simulink model "scenario"  (R2022a)
settings: Solver=FixedStepDiscrete  StartTime=0.0  StopTime=200  RelTol=1e-3
model workspace (MAT data in the model file):
  firstWarning = 1
  originalScenarioChecksum = '4DD51816F7E71EE9C2F131BDCC6CE010'
undefined symbols (not defined in the file or in its folder): driving
libraries: drivingscenarioandsensors x4
settings Model: Creator=giovanni02  LastModifiedBy=giovanni02

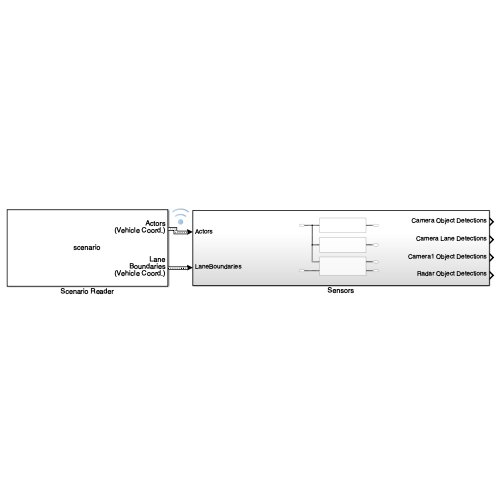
[thumbnail: Simulink's stored preview of the top-level diagram]
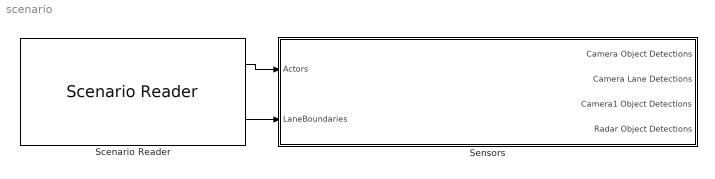
== system scenario ==
  Scenario Reader : drivingscenarioandsensors/Scenario Reader  ScenarioSource=From file  ScenarioFileName=/Users/giovanni02/Desktop/Progetti/HybridRL/scenario.mat  ScenarioVariableName=scenario  OutputCoordinateSystem=Vehicle coordinates  EgoVehicleSource=Scenario  EgoVehicleActorID=1  OrientVehiclesOnRoad=off  OutputEgoVehiclePose=off  OutputEgoVehicleState=off  SampleTime=0.1  LaneBoundaryOutput=Ego vehicle lane boundaries  LaneBoundaryDistance=linspace(-150, 150, 101)  LaneBoundaryLocation=Center of lane markings  BusNameSource=Auto  BusName=BusActors  BusNumActorsSource=Scenario  BusNumActors=100  BusName2Source=Auto  BusName2=BusLaneBoundaries  BusNumLaneBoundariesSource=Scenario  BusNumLaneBoundaries=10  BusName3Source=Auto  BusName3=BusEgoActor  BusName4Source=Auto  BusName4=BusEgoState  ShowCoordinateLabels=on  SimulateUsing=Interpreted execution
  Sensors : Subsystem
  wires:
  Scenario Reader/1 -> Sensors/1(Actors)
  Scenario Reader/2 -> Sensors/2(LaneBoundaries)

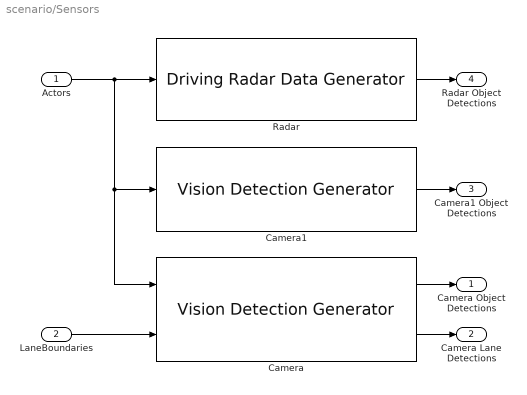
== system scenario/Sensors ==
  Actors : Inport
  LaneBoundaries : Inport  Port=2
  Camera : drivingscenarioandsensors/Vision Detection Generator  SensorIndex=1  DetectorOutput=Lanes and objects  UpdateInterval=0.1  LaneUpdateInterval=0.1  SensorLocation=[1.9 0]  Height=1.1  Yaw=0  Pitch=1  Roll=0  BusNameSource=Auto  BusName=BusObjectDetections  BusName2Source=Auto  BusName2=BusLaneDetections  MaxNumDetectionsSource=Property  MaxNumDetections=50  MaxNumLanesSource=Property  MaxNumLanes=30  DetectionCoordinates=Ego Cartesian  SimulateUsing=Interpreted execution  MaxRange=150  BoundingBoxAccuracy=5  ProcessNoiseIntensity=5  MaxSpeed=100  MaxAllowedOcclusion=0.5  MinObjectImageSize=[15 15]  DetectionProbability=0.9  FalsePositivesPerImage=0.1  MinLaneImageSize=[20 3]  LaneBoundaryAccuracy=3  HasNoise=on  InitialSeedSource=Repeatable  InitialSeed=0  UsedSeed=0  ActorProfilesSource=From Scenario Reader block  ActorProfilesParameters=driving.internal.ActorProfilesParameters  ActorProfilesExpression=[struct('ActorID',1,'ClassID',1,'Length',4.848,'Width',1.842,'Height',1.517,'OriginOffset',[-1.305 0 0],'MeshVertices',[3.729 0.921 0.929096885813149;3.729 -0.921 0.929096885813149;3.729 -0.921 0.341193771626297;3.729 0.921 0.341193771626297;3.729 0.921 0.929096885813149;2.517 0.921 1.07607266435986;2.517 -0.921 1.07607266435986;3.729 -0.921 0.929096885813149;1.7898 0.7368 1.517;0.3354 0.7368 1.517;0.3354 -0.7368 1.517;1.7898 -0.7368 1.517;-0.3918 0.921 1.07607266435986;-1.119 0.921 0.929096885813149;-1.119 -0.921 0.929096885813149;-0.3918 -0.921 1.07607266435986;3.729 0.921 0.929096885813149;3.729 0.921 0.341193771626297;2.517 0.921 0.341193771626297;2.517 0.921 1.07607266435986;2.517 0.921 1.07607266435986;2.517 0.921 0.341193771626297;-0.3918 0.921 0.341193771626297;-0.3918 0.921 1.07607266435986;-0.3918 0.921 1.07607266435986;-0.3918 0.921 0.341193771626297;-1.119 0.921 0.385286505190311;-1.119 0.921 0.929096885813149;2.517 0.921 1.07607266435986;-0.3918 0.921 1.07607266435986;0.3354 0.7368 1.517;1.7898 0.7368 1.517;3.729 -0.921 0.929096885813149;3.729 -0.921 0.341193771626297;2.517 -0.921 0.341193771626297;2.517 -0.921 1.07607266435986;2.517 -0.921 1.07607266435986;2.517 -0.921 0.341193771626297;-0.3918 -0.921 0.341193771626297;-0.3918 -0.921 1.07607266435986;-0.3918 -0.921 1.07607266435986;-0.3918 -0.921 0.341193771626297;-1.119 -0.921 0.385286505190311;-1.119 -0.921 0.929096885813149;2.517 -0.921 1.07607266435986;-0.3918 -0.921 1.07607266435986;0.3354 -0.7368 1.517;1.7898 -0.7368 1.517;-0.3918 0.921 1.07607266435986;-0.3918 -0.921 1.07607266435986;0.3354 -0.7368 1.517;0.3354 0.7368 1.517;2.517 -0.921 1.07607266435986;1.7898 -0.7368 1.517;1.7898 0.7368 1.517;2.517 0.921 1.07607266435986;-1.119 0.921 0.929096885813149;-1.119 0.921 0.385286505190311;-1.119 -0.921 0.385286505190311;-1.119 -0.921 0.929096885813149;3.729 0.921 0.341193771626297;3.729 -0.921 0.341193771626297;-0.3918 -0.921 0.341193771626297;-0.3918 0.921 0.341193771626297;-0.3918 0.921 0.341193771626297;-1.119 0.921 0.385286505190311;-1.119 -0.921 0.385286505190311;-0.3918 -0.921 0.341193771626297;-0.0875106382978725 -0.6447 0;-0.0875106382978725 -0.8903 0;0.109534987981281 -0.6447 0.065162212005738;0.109534987981281 -0.8903 0.065162212005738;0.231315882356307 -0.6447 0.235759097818887;0.231315882356307 -0.8903 0.235759097818887;0.231315882356307 -0.6447 0.446628445433708;0.231315882356307 -0.8903 0.446628445433708;0.109534987981281 -0.6447 0.617225331246857;0.109534987981281 -0.8903 0.617225331246857;-0.0875106382978725 -0.6447 0.682387543252595;-0.0875106382978725 -0.8903 0.682387543252595;-0.284556264577026 -0.6447 0.617225331246857;-0.284556264577026 -0.8903 0.617225331246857;-0.406337158952052 -0.6447 0.446628445433708;-0.406337158952052 -0.8903 0.446628445433708;-0.406337158952052 -0.6447 0.235759097818887;-0.406337158952052 -0.8903 0.235759097818887;-0.284556264577026 -0.6447 0.065162212005738;-0.284556264577026 -0.8903 0.065162212005738;-0.0875106382978725 -0.6447 0;-0.0875106382978725 -0.8903 0;-0.0875106382978725 -0.6447 0;0.109534987981281 -0.6447 0.065162212005738;0.231315882356307 -0.6447 0.235759097818887;0.231315882356307 -0.6447 0.446628445433708;0.109534987981281 -0.6447 0.617225331246857;-0.0875106382978725 -0.6447 0.682387543252595;-0.284556264577026 -0.6447 0.617225331246857;-0.406337158952052 -0.6447 0.446628445433708;-0.406337158952052 -0.6447 0.235759097818887;-0.284556264577026 -0.6447 0.065162212005738;-0.0875106382978725 -0.8903 0;0.109534987981281 -0.8903 0.065162212005738;0.231315882356307 -0.8903 0.235759097818887;0.231315882356307 -0.8903 0.446628445433708;0.109534987981281 -0.8903 0.617225331246857;-0.0875106382978725 -0.8903 0.682387543252595;-0.284556264577026 -0.8903 0.617225331246857;-0.406337158952052 -0.8903 0.446628445433708;-0.406337158952052 -0.8903 0.235759097818887;-0.284556264577026 -0.8903 0.065162212005738;-0.0875106382978725 0.8903 0;-0.0875106382978725 0.6447 0;0.109534987981281 0.8903 0.065162212005738;0.109534987981281 0.6447 0.065162212005738;0.231315882356307 0.8903 0.235759097818887;0.231315882356307 0.6447 ...(+4912 chars)],'MeshFaces',[1 2 3;3 4 1;5 6 7;7 8 5;9 10 11;11 12 9;13 14 15;15 16 13;17 18 19;19 20 17;21 22 23;23 24 21;25 26 27;27 28 25;29 30 31;31 32 29;33 34 35;35 36 33;37 38 39;39 40 37;41 42 43;43 44 41;45 46 47;47 48 45;49 50 51;51 52 49;53 54 55;55 56 53;57 58 59;59 60 57;61 62 63;63 64 61;65 66 67;67 68 65;69 71 72;72 70 69;71 73 74;74 72 71;73 75 76;76 74 73;75 77 78;78 76 75;77 79 80;80 78 77;79 81 82;82 80 79;81 83 84;84 82 81;83 85 86;86 84 83;85 87 88;88 86 85;87 89 90;90 88 87;91 92 93;91 93 94;91 94 95;91 95 96;91 96 97;91 97 98;91 98 99;91 99 100;101 102 103;101 103 104;101 104 105;101 105 106;101 106 107;101 107 108;101 108 109;101 109 110;111 113 114;114 112 111;113 115 116;116 114 113;115 117 118;118 116 115;117 119 120;120 118 117;119 121 122;122 120 119;121 123 124;124 122 121;123 125 126;126 124 123;125 127 128;128 126 125;127 129 130;130 128 127;129 131 132;132 130 129;133 134 135;133 135 136;133 136 137;133 137 138;133 138 139;133 139 140;133 140 141;133 141 142;143 144 145;143 145 146;143 146 147;143 147 148;143 148 149;143 149 150;143 150 151;143 151 152;153 155 156;156 154 153;155 157 158;158 156 155;157 159 160;160 158 157;159 161 162;162 160 159;161 163 164;164 162 161;163 165 166;166 164 163;165 167 168;168 166 165;167 169 170;170 168 167;169 171 172;172 170 169;171 173 174;174 172 171;175 176 177;175 177 178;175 178 179;175 179 180;175 180 181;175 181 182;175 182 183;175 183 184;185 186 187;185 187 188;185 188 189;185 189 190;185 190 191;185 191 192;185 192 193;185 193 194;195 197 198;198 196 195;197 199 200;200 198 197;199 201 202;202 200 199;201 203 204;204 202 201;203 205 206;206 204 203;205 207 208;208 206 205;207 209 210;210 208 207;209 211 212;212 210 209;211 213 214;214 212 211;213 215 216;216 214 213;217 218 219;217 219 220;217 220 221;217 221 222;217 222 223;217 223 224;217 224 225;217 225 226;227 228 229;227 229 230;227 230 231;227 231 232;227 232 233;227 233 234;227 234 235;227 235 236],'RCSPattern',[10 10;10 10],'RCSAzimuthAngles',[-180 180],'RCSElevationAngles',[-90 90])]  Intrinsics=driving.internal.cameraIntrinsics('FocalLength',[800 800],'PrincipalPoint',[400 240],'ImageSize',[500 700],'RadialDistortion',[0 0],'TangentialDistortion',[0 0],'Skew',0)
  Camera1 : drivingscenarioandsensors/Vision Detection Generator  SensorIndex=2  DetectorOutput=Objects only  UpdateInterval=0.1  LaneUpdateInterval=0.1  SensorLocation=[-1 0]  Height=1.1  Yaw=-180  Pitch=1  Roll=0  BusNameSource=Auto  BusName=BusObjectDetections  BusName2Source=Auto  BusName2=BusLaneDetections  MaxNumDetectionsSource=Property  MaxNumDetections=50  MaxNumLanesSource=Property  MaxNumLanes=30  DetectionCoordinates=Ego Cartesian  SimulateUsing=Interpreted execution  MaxRange=100  BoundingBoxAccuracy=5  ProcessNoiseIntensity=5  MaxSpeed=100  MaxAllowedOcclusion=0.5  MinObjectImageSize=[15 15]  DetectionProbability=0.9  FalsePositivesPerImage=0.1  MinLaneImageSize=[20 3]  LaneBoundaryAccuracy=3  HasNoise=on  InitialSeedSource=Repeatable  InitialSeed=0  UsedSeed=0  ActorProfilesSource=From Scenario Reader block  ActorProfilesParameters=driving.internal.ActorProfilesParameters  ActorProfilesExpression=[struct('ActorID',1,'ClassID',1,'Length',4.848,'Width',1.842,'Height',1.517,'OriginOffset',[-1.305 0 0],'MeshVertices',[3.729 0.921 0.929096885813149;3.729 -0.921 0.929096885813149;3.729 -0.921 0.341193771626297;3.729 0.921 0.341193771626297;3.729 0.921 0.929096885813149;2.517 0.921 1.07607266435986;2.517 -0.921 1.07607266435986;3.729 -0.921 0.929096885813149;1.7898 0.7368 1.517;0.3354 0.7368 1.517;0.3354 -0.7368 1.517;1.7898 -0.7368 1.517;-0.3918 0.921 1.07607266435986;-1.119 0.921 0.929096885813149;-1.119 -0.921 0.929096885813149;-0.3918 -0.921 1.07607266435986;3.729 0.921 0.929096885813149;3.729 0.921 0.341193771626297;2.517 0.921 0.341193771626297;2.517 0.921 1.07607266435986;2.517 0.921 1.07607266435986;2.517 0.921 0.341193771626297;-0.3918 0.921 0.341193771626297;-0.3918 0.921 1.07607266435986;-0.3918 0.921 1.07607266435986;-0.3918 0.921 0.341193771626297;-1.119 0.921 0.385286505190311;-1.119 0.921 0.929096885813149;2.517 0.921 1.07607266435986;-0.3918 0.921 1.07607266435986;0.3354 0.7368 1.517;1.7898 0.7368 1.517;3.729 -0.921 0.929096885813149;3.729 -0.921 0.341193771626297;2.517 -0.921 0.341193771626297;2.517 -0.921 1.07607266435986;2.517 -0.921 1.07607266435986;2.517 -0.921 0.341193771626297;-0.3918 -0.921 0.341193771626297;-0.3918 -0.921 1.07607266435986;-0.3918 -0.921 1.07607266435986;-0.3918 -0.921 0.341193771626297;-1.119 -0.921 0.385286505190311;-1.119 -0.921 0.929096885813149;2.517 -0.921 1.07607266435986;-0.3918 -0.921 1.07607266435986;0.3354 -0.7368 1.517;1.7898 -0.7368 1.517;-0.3918 0.921 1.07607266435986;-0.3918 -0.921 1.07607266435986;0.3354 -0.7368 1.517;0.3354 0.7368 1.517;2.517 -0.921 1.07607266435986;1.7898 -0.7368 1.517;1.7898 0.7368 1.517;2.517 0.921 1.07607266435986;-1.119 0.921 0.929096885813149;-1.119 0.921 0.385286505190311;-1.119 -0.921 0.385286505190311;-1.119 -0.921 0.929096885813149;3.729 0.921 0.341193771626297;3.729 -0.921 0.341193771626297;-0.3918 -0.921 0.341193771626297;-0.3918 0.921 0.341193771626297;-0.3918 0.921 0.341193771626297;-1.119 0.921 0.385286505190311;-1.119 -0.921 0.385286505190311;-0.3918 -0.921 0.341193771626297;-0.0875106382978725 -0.6447 0;-0.0875106382978725 -0.8903 0;0.109534987981281 -0.6447 0.065162212005738;0.109534987981281 -0.8903 0.065162212005738;0.231315882356307 -0.6447 0.235759097818887;0.231315882356307 -0.8903 0.235759097818887;0.231315882356307 -0.6447 0.446628445433708;0.231315882356307 -0.8903 0.446628445433708;0.109534987981281 -0.6447 0.617225331246857;0.109534987981281 -0.8903 0.617225331246857;-0.0875106382978725 -0.6447 0.682387543252595;-0.0875106382978725 -0.8903 0.682387543252595;-0.284556264577026 -0.6447 0.617225331246857;-0.284556264577026 -0.8903 0.617225331246857;-0.406337158952052 -0.6447 0.446628445433708;-0.406337158952052 -0.8903 0.446628445433708;-0.406337158952052 -0.6447 0.235759097818887;-0.406337158952052 -0.8903 0.235759097818887;-0.284556264577026 -0.6447 0.065162212005738;-0.284556264577026 -0.8903 0.065162212005738;-0.0875106382978725 -0.6447 0;-0.0875106382978725 -0.8903 0;-0.0875106382978725 -0.6447 0;0.109534987981281 -0.6447 0.065162212005738;0.231315882356307 -0.6447 0.235759097818887;0.231315882356307 -0.6447 0.446628445433708;0.109534987981281 -0.6447 0.617225331246857;-0.0875106382978725 -0.6447 0.682387543252595;-0.284556264577026 -0.6447 0.617225331246857;-0.406337158952052 -0.6447 0.446628445433708;-0.406337158952052 -0.6447 0.235759097818887;-0.284556264577026 -0.6447 0.065162212005738;-0.0875106382978725 -0.8903 0;0.109534987981281 -0.8903 0.065162212005738;0.231315882356307 -0.8903 0.235759097818887;0.231315882356307 -0.8903 0.446628445433708;0.109534987981281 -0.8903 0.617225331246857;-0.0875106382978725 -0.8903 0.682387543252595;-0.284556264577026 -0.8903 0.617225331246857;-0.406337158952052 -0.8903 0.446628445433708;-0.406337158952052 -0.8903 0.235759097818887;-0.284556264577026 -0.8903 0.065162212005738;-0.0875106382978725 0.8903 0;-0.0875106382978725 0.6447 0;0.109534987981281 0.8903 0.065162212005738;0.109534987981281 0.6447 0.065162212005738;0.231315882356307 0.8903 0.235759097818887;0.231315882356307 0.6447 ...(+4912 chars)],'MeshFaces',[1 2 3;3 4 1;5 6 7;7 8 5;9 10 11;11 12 9;13 14 15;15 16 13;17 18 19;19 20 17;21 22 23;23 24 21;25 26 27;27 28 25;29 30 31;31 32 29;33 34 35;35 36 33;37 38 39;39 40 37;41 42 43;43 44 41;45 46 47;47 48 45;49 50 51;51 52 49;53 54 55;55 56 53;57 58 59;59 60 57;61 62 63;63 64 61;65 66 67;67 68 65;69 71 72;72 70 69;71 73 74;74 72 71;73 75 76;76 74 73;75 77 78;78 76 75;77 79 80;80 78 77;79 81 82;82 80 79;81 83 84;84 82 81;83 85 86;86 84 83;85 87 88;88 86 85;87 89 90;90 88 87;91 92 93;91 93 94;91 94 95;91 95 96;91 96 97;91 97 98;91 98 99;91 99 100;101 102 103;101 103 104;101 104 105;101 105 106;101 106 107;101 107 108;101 108 109;101 109 110;111 113 114;114 112 111;113 115 116;116 114 113;115 117 118;118 116 115;117 119 120;120 118 117;119 121 122;122 120 119;121 123 124;124 122 121;123 125 126;126 124 123;125 127 128;128 126 125;127 129 130;130 128 127;129 131 132;132 130 129;133 134 135;133 135 136;133 136 137;133 137 138;133 138 139;133 139 140;133 140 141;133 141 142;143 144 145;143 145 146;143 146 147;143 147 148;143 148 149;143 149 150;143 150 151;143 151 152;153 155 156;156 154 153;155 157 158;158 156 155;157 159 160;160 158 157;159 161 162;162 160 159;161 163 164;164 162 161;163 165 166;166 164 163;165 167 168;168 166 165;167 169 170;170 168 167;169 171 172;172 170 169;171 173 174;174 172 171;175 176 177;175 177 178;175 178 179;175 179 180;175 180 181;175 181 182;175 182 183;175 183 184;185 186 187;185 187 188;185 188 189;185 189 190;185 190 191;185 191 192;185 192 193;185 193 194;195 197 198;198 196 195;197 199 200;200 198 197;199 201 202;202 200 199;201 203 204;204 202 201;203 205 206;206 204 203;205 207 208;208 206 205;207 209 210;210 208 207;209 211 212;212 210 209;211 213 214;214 212 211;213 215 216;216 214 213;217 218 219;217 219 220;217 220 221;217 221 222;217 222 223;217 223 224;217 224 225;217 225 226;227 228 229;227 229 230;227 230 231;227 231 232;227 232 233;227 233 234;227 234 235;227 235 236],'RCSPattern',[10 10;10 10],'RCSAzimuthAngles',[-180 180],'RCSElevationAngles',[-90 90])]  Intrinsics=driving.internal.cameraIntrinsics('FocalLength',[1814.81018227767 1814.81018227767],'PrincipalPoint',[320 240],'ImageSize',[480 640],'RadialDistortion',[0 0],'TangentialDistortion',[0 0],'Skew',0)
  Radar : drivingscenarioandsensors/Driving Radar Data Generator  SensorIndex=3  UpdateRate=10  MountingLocation=[3.7 0 0.2]  MountingAngles=[0 0 0]  HasElevation=off  HasRangeRate=on  HasNoise=on  HasFalseAlarms=on  HasOcclusion=on  MaxNumReportsSource=Property  MaxNumReports=50  TargetReportFormat=Detections  DetectionCoordinates=Body  TrackCoordinates=Body  BusNameSource=Auto  BusName=BusDrivingRadarDataGenerator  AzimuthResolution=4  ElevationResolution=5  RangeResolution=2.5  RangeRateResolution=0.5  AzimuthBiasFraction=0.1  ElevationBiasFraction=0.1  RangeBiasFraction=0.05  RangeRateBiasFraction=0.05  FieldOfView=[20 5]  RangeLimits=[0 100]  RangeRateLimits=[-100 100]  DetectionProbability=0.9  FalseAlarmRate=1e-06  ReferenceRange=100  ReferenceRCS=0  CenterFrequency=77000000000  FilterInitializationFcn=initcvekf  ConfirmationThreshold=[2 3]  DeletionThreshold=[5 5]  InitialSeedSource=Repeatable  InitialSeed=0  UsedSeed=0  ProfilesSource=Parameters  ProfilesParameters=driving.internal.ActorProfilesRadarParameters  ProfilesExpression=[struct('ActorID',1,'ClassID',1,'Length',4.848,'Width',1.842,'Height',1.517,'OriginOffset',[-1.305 0 0],'MeshVertices',[3.729 0.921 0.929096885813149;3.729 -0.921 0.929096885813149;3.729 -0.921 0.341193771626297;3.729 0.921 0.341193771626297;3.729 0.921 0.929096885813149;2.517 0.921 1.07607266435986;2.517 -0.921 1.07607266435986;3.729 -0.921 0.929096885813149;1.7898 0.7368 1.517;0.3354 0.7368 1.517;0.3354 -0.7368 1.517;1.7898 -0.7368 1.517;-0.3918 0.921 1.07607266435986;-1.119 0.921 0.929096885813149;-1.119 -0.921 0.929096885813149;-0.3918 -0.921 1.07607266435986;3.729 0.921 0.929096885813149;3.729 0.921 0.341193771626297;2.517 0.921 0.341193771626297;2.517 0.921 1.07607266435986;2.517 0.921 1.07607266435986;2.517 0.921 0.341193771626297;-0.3918 0.921 0.341193771626297;-0.3918 0.921 1.07607266435986;-0.3918 0.921 1.07607266435986;-0.3918 0.921 0.341193771626297;-1.119 0.921 0.385286505190311;-1.119 0.921 0.929096885813149;2.517 0.921 1.07607266435986;-0.3918 0.921 1.07607266435986;0.3354 0.7368 1.517;1.7898 0.7368 1.517;3.729 -0.921 0.929096885813149;3.729 -0.921 0.341193771626297;2.517 -0.921 0.341193771626297;2.517 -0.921 1.07607266435986;2.517 -0.921 1.07607266435986;2.517 -0.921 0.341193771626297;-0.3918 -0.921 0.341193771626297;-0.3918 -0.921 1.07607266435986;-0.3918 -0.921 1.07607266435986;-0.3918 -0.921 0.341193771626297;-1.119 -0.921 0.385286505190311;-1.119 -0.921 0.929096885813149;2.517 -0.921 1.07607266435986;-0.3918 -0.921 1.07607266435986;0.3354 -0.7368 1.517;1.7898 -0.7368 1.517;-0.3918 0.921 1.07607266435986;-0.3918 -0.921 1.07607266435986;0.3354 -0.7368 1.517;0.3354 0.7368 1.517;2.517 -0.921 1.07607266435986;1.7898 -0.7368 1.517;1.7898 0.7368 1.517;2.517 0.921 1.07607266435986;-1.119 0.921 0.929096885813149;-1.119 0.921 0.385286505190311;-1.119 -0.921 0.385286505190311;-1.119 -0.921 0.929096885813149;3.729 0.921 0.341193771626297;3.729 -0.921 0.341193771626297;-0.3918 -0.921 0.341193771626297;-0.3918 0.921 0.341193771626297;-0.3918 0.921 0.341193771626297;-1.119 0.921 0.385286505190311;-1.119 -0.921 0.385286505190311;-0.3918 -0.921 0.341193771626297;-0.0875106382978725 -0.6447 0;-0.0875106382978725 -0.8903 0;0.109534987981281 -0.6447 0.065162212005738;0.109534987981281 -0.8903 0.065162212005738;0.231315882356307 -0.6447 0.235759097818887;0.231315882356307 -0.8903 0.235759097818887;0.231315882356307 -0.6447 0.446628445433708;0.231315882356307 -0.8903 0.446628445433708;0.109534987981281 -0.6447 0.617225331246857;0.109534987981281 -0.8903 0.617225331246857;-0.0875106382978725 -0.6447 0.682387543252595;-0.0875106382978725 -0.8903 0.682387543252595;-0.284556264577026 -0.6447 0.617225331246857;-0.284556264577026 -0.8903 0.617225331246857;-0.406337158952052 -0.6447 0.446628445433708;-0.406337158952052 -0.8903 0.446628445433708;-0.406337158952052 -0.6447 0.235759097818887;-0.406337158952052 -0.8903 0.235759097818887;-0.284556264577026 -0.6447 0.065162212005738;-0.284556264577026 -0.8903 0.065162212005738;-0.0875106382978725 -0.6447 0;-0.0875106382978725 -0.8903 0;-0.0875106382978725 -0.6447 0;0.109534987981281 -0.6447 0.065162212005738;0.231315882356307 -0.6447 0.235759097818887;0.231315882356307 -0.6447 0.446628445433708;0.109534987981281 -0.6447 0.617225331246857;-0.0875106382978725 -0.6447 0.682387543252595;-0.284556264577026 -0.6447 0.617225331246857;-0.406337158952052 -0.6447 0.446628445433708;-0.406337158952052 -0.6447 0.235759097818887;-0.284556264577026 -0.6447 0.065162212005738;-0.0875106382978725 -0.8903 0;0.109534987981281 -0.8903 0.065162212005738;0.231315882356307 -0.8903 0.235759097818887;0.231315882356307 -0.8903 0.446628445433708;0.109534987981281 -0.8903 0.617225331246857;-0.0875106382978725 -0.8903 0.682387543252595;-0.284556264577026 -0.8903 0.617225331246857;-0.406337158952052 -0.8903 0.446628445433708;-0.406337158952052 -0.8903 0.235759097818887;-0.284556264577026 -0.8903 0.065162212005738;-0.0875106382978725 0.8903 0;-0.0875106382978725 0.6447 0;0.109534987981281 0.8903 0.065162212005738;0.109534987981281 0.6447 0.065162212005738;0.231315882356307 0.8903 0.235759097818887;0.231315882356307 0.6447 ...(+4912 chars)],'MeshFaces',[1 2 3;3 4 1;5 6 7;7 8 5;9 10 11;11 12 9;13 14 15;15 16 13;17 18 19;19 20 17;21 22 23;23 24 21;25 26 27;27 28 25;29 30 31;31 32 29;33 34 35;35 36 33;37 38 39;39 40 37;41 42 43;43 44 41;45 46 47;47 48 45;49 50 51;51 52 49;53 54 55;55 56 53;57 58 59;59 60 57;61 62 63;63 64 61;65 66 67;67 68 65;69 71 72;72 70 69;71 73 74;74 72 71;73 75 76;76 74 73;75 77 78;78 76 75;77 79 80;80 78 77;79 81 82;82 80 79;81 83 84;84 82 81;83 85 86;86 84 83;85 87 88;88 86 85;87 89 90;90 88 87;91 92 93;91 93 94;91 94 95;91 95 96;91 96 97;91 97 98;91 98 99;91 99 100;101 102 103;101 103 104;101 104 105;101 105 106;101 106 107;101 107 108;101 108 109;101 109 110;111 113 114;114 112 111;113 115 116;116 114 113;115 117 118;118 116 115;117 119 120;120 118 117;119 121 122;122 120 119;121 123 124;124 122 121;123 125 126;126 124 123;125 127 128;128 126 125;127 129 130;130 128 127;129 131 132;132 130 129;133 134 135;133 135 136;133 136 137;133 137 138;133 138 139;133 139 140;133 140 141;133 141 142;143 144 145;143 145 146;143 146 147;143 147 148;143 148 149;143 149 150;143 150 151;143 151 152;153 155 156;156 154 153;155 157 158;158 156 155;157 159 160;160 158 157;159 161 162;162 160 159;161 163 164;164 162 161;163 165 166;166 164 163;165 167 168;168 166 165;167 169 170;170 168 167;169 171 172;172 170 169;171 173 174;174 172 171;175 176 177;175 177 178;175 178 179;175 179 180;175 180 181;175 181 182;175 182 183;175 183 184;185 186 187;185 187 188;185 188 189;185 189 190;185 190 191;185 191 192;185 192 193;185 193 194;195 197 198;198 196 195;197 199 200;200 198 197;199 201 202;202 200 199;201 203 204;204 202 201;203 205 206;206 204 203;205 207 208;208 206 205;207 209 210;210 208 207;209 211 212;212 210 209;211 213 214;214 212 211;213 215 216;216 214 213;217 218 219;217 219 220;217 220 221;217 221 222;217 222 223;217 223 224;217 224 225;217 225 226;227 228 229;227 229 230;227 230 231;227 231 232;227 232 233;227 233 234;227 234 235;227 235 236],'RCSPattern',[10 10;10 10],'RCSAzimuthAngles',[-180 180],'RCSElevationAngles',[-90 90])]
      settings: SourceProductBaseCode=DR
  Camera Object Detections : Outport
  Camera Lane Detections : Outport  Port=2
  Camera1 Object Detections : Outport  Port=3
  Radar Object Detections : Outport  Port=4
  wires:
  Actors/1 -> Camera1/1, Camera/1, Radar/1
  Camera1/1 -> Camera1 Object Detections/1
  Camera/1 -> Camera Object Detections/1
  Radar/1 -> Radar Object Detections/1
  LaneBoundaries/1 -> Camera/2
  Camera/2 -> Camera Lane Detections/1
